simulink model "Single_Phase_Pulse_Width_Modulated_Inverter"  (R2020b)
settings: Solver=VariableStepAuto  StartTime=0.0  StopTime=1  RelTol=1e-3
libraries: powerlib x9, simulink x1, powerlib_meascontrol x1
settings Model: Creator=adima  LastModifiedBy=adima

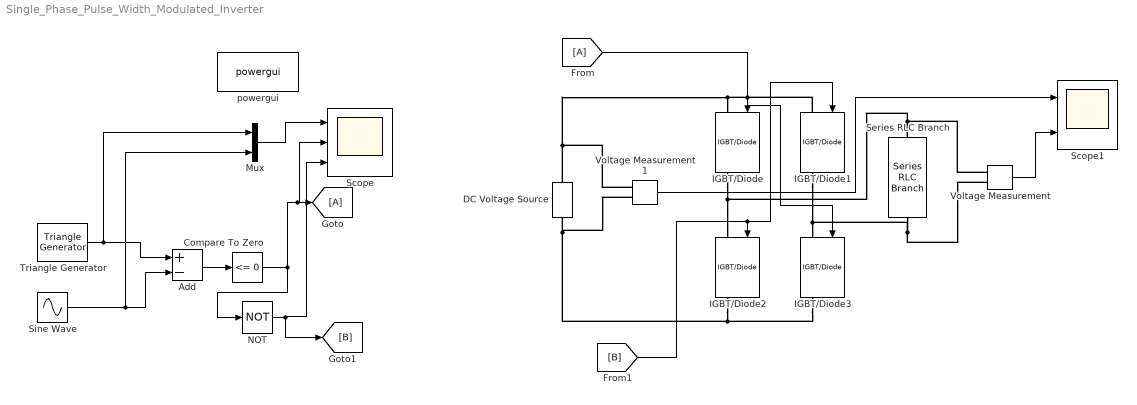
== system Single_Phase_Pulse_Width_Modulated_Inverter ==
  Add : Sum  Inputs=+-
  Compare To Zero : simulink/Logic and Bit Operations/Compare To Zero  relop=<=  OutDataTypeStr=boolean
  DC Voltage Source : powerlib/Electrical Sources/DC Voltage Source  Amplitude=100  Measurements=None
  IGBT/Diode{,1..3} (4 alike) : powerlib/Power Electronics/IGBT//Diode  Ron=1e-3  Rs=1e5  Cs=inf  Measurements=on
  Mux : Mux  Inputs=2
  NOT : Logic  Operator=NOT  IconShape=distinctive  AllPortsSameDT=off  OutDataTypeStr=boolean
  Scope : Scope  NumInputPorts=3
  Scope1 : Scope  NumInputPorts=2
  Series RLC Branch : powerlib/Elements/Series RLC Branch  LConnTagsString=__new0  RConnTagsString=__new0  BranchType=R  Resistance=1  Inductance=1e-3  SetiL0=off  InitialCurrent=0  Capacitance=1e-6  Setx0=off  InitialVoltage=0  Measurements=None
  Sine Wave : Sin  Frequency=2*pi*50  SampleTime=0
  Triangle Generator : powerlib_meascontrol/Pulse & Signal Generators/Triangle Generator  Freq=1e3  Phase=90  Ts=0
  Voltage Measurement : powerlib/Measurements/Voltage Measurement  PhasorSimulation=off  OutputType=Complex  PSBequivalent=0
  Voltage Measurement1 : powerlib/Measurements/Voltage Measurement  PhasorSimulation=off  OutputType=Complex  PSBequivalent=0
  powergui : powerlib/powergui  Priority=1  SimulationMode=Continuous  SampleTime=50e-6  frequency=60  Iterations=50  frequencyindice=0  Pbase=100e6  ErrMax=1e-4  UnitsV=kV  UnitsW=MW  buscounter=0  FunctionMessages=off  echomessages=off  EnableUseOfTLC=off  CurrentSourceSwitches=off  DisableSnubberDevices=off  DisableRonSwitches=off  DisableVfSwitches=off  DisplayEquations=off  AutomaticDiscreteSolvers=off  SolverType=Tustin/Backward Euler (TBE)  Interpol=off  ExternalGateDelay=off  methode=off  Ts=100  x0status=blocks  SPID=on  SwTol=0  HookPort=off  NonlinearTolerance=1e-4  nMaxIteration=100  ContinueOnMaxIteration=off  RestoreLinks=warning  ResistiveCurrentMeasurement=off  Frange=[0:2:500]  Ylog=off  Xlog=on  ShowGrid=off  save=off  variable=ZData  structure=0  ZoomFFT=off  StartTime=0.0  cycles=1  DisplayStyle=1  fundamental=60  FreqAxis=off  MaxFrequency=1000  frequencyindicesteady=1  RmsSteady=1  display=off
  wires:
  Triangle Generator/1 -> Mux/1, Add/1
  Sine Wave/1 -> Mux/2, Add/2
  Add/1 -> Compare To Zero/1
  Compare To Zero/1 -> NOT/1, Scope/2, [A]
  NOT/1 -> Scope/3, [B]
  Mux/1 -> Scope/1
  [A] -> IGBT/Diode3/1, IGBT/Diode/1
  [B] -> IGBT/Diode1/1, IGBT/Diode2/1
  Voltage Measurement/1 -> Scope1/2
  Voltage Measurement1/1 -> Scope1/1
  connections:
  DC Voltage Source/RConn1 -- Voltage Measurement1/LConn1 -- IGBT/Diode1/LConn1 -- IGBT/Diode/LConn1
  IGBT/Diode2/RConn1 -- Voltage Measurement1/LConn2 -- DC Voltage Source/LConn1 -- IGBT/Diode3/RConn1
  IGBT/Diode/RConn1 -- Voltage Measurement/LConn1 -- Series RLC Branch/LConn1 -- IGBT/Diode2/LConn1
  IGBT/Diode1/RConn1 -- Voltage Measurement/LConn2 -- Series RLC Branch/RConn1 -- IGBT/Diode3/LConn1
